simulink library "control_design_lib"  (Simulink 7.1)
libraries: control_design_lib x1
settings Model: Creator=jporter  LastModifiedBy=jporter

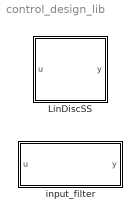
== system control_design_lib ==
  LinDiscSS : Subsystem  mask(Linear Discrete State Space){Add=0, Bdd=0, Cdd=0, Ddd=0, x0=0, Tsamp=0}
      mask prompts: Add "Ad"; Bdd "Bd"; Cdd "Cd"; Ddd "Dd"; x0 "Initial condition:"; Tsamp "Sample time:"
      mask help:
      | Implements a linear discrete state-space filter using blocks
      | which are compatible with the HCDDES toolchain code generator.
  input_filter : Subsystem  mask{wn=1, zeta=0.9, Tsamp=0.02}
      mask prompts: wn "omega_n"; Tsamp "Sample time"
      mask init:
      | Fsys = tf([wn^2],[1,2*zeta*wn,wn^2]);
      | Fd = c2d( Fsys, Tsamp, 'zoh' );
      | FS = ss( Fd );
      | Add = FS.a;
      | Bdd = FS.b;
      | Cdd = FS.c;
      | Ddd = FS.d;

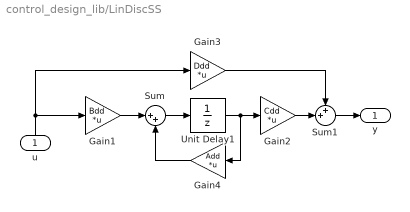
== system control_design_lib/LinDiscSS ==
  u : Inport  Orientation=up
  Gain1 : Gain  Gain=Bdd  Multiplication=Matrix(K*u)  ParameterDataType=sfix(16)  ParameterScaling=2^0  OutDataType=sfix(16)  OutScaling=2^0
  Gain2 : Gain  Gain=Cdd  Multiplication=Matrix(K*u) (u vector)  ParameterDataType=sfix(16)  ParameterScaling=2^0  OutDataType=sfix(16)  OutScaling=2^0
  Gain3 : Gain  Gain=Ddd  Multiplication=Matrix(K*u)  ParameterDataType=sfix(16)  ParameterScaling=2^0  OutDataType=sfix(16)  OutScaling=2^0
  Gain4 : Gain  Orientation=left  Gain=Add  Multiplication=Matrix(K*u) (u vector)  ParameterDataType=sfix(16)  ParameterScaling=2^0  OutDataType=sfix(16)  OutScaling=2^0
  Sum : Sum  Inputs=|++  OutDataType=sfix(16)  OutScaling=2^0
  Sum1 : Sum  Inputs=++|  OutDataType=sfix(16)  OutScaling=2^0
  Unit Delay1 : UnitDelay  X0=x0  SampleTime=Tsamp
  y : Outport
  wires:
  Gain1/1 -> Sum/1
  Gain3/1 -> Sum1/1
  Gain2/1 -> Sum1/2
  Sum/1 -> Unit Delay1/1
  Unit Delay1/1 -> Gain2/1, Gain4/1
  Gain4/1 -> Sum/2
  u/1 -> Gain1/1, Gain3/1
  Sum1/1 -> y/1

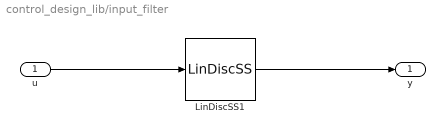
== system control_design_lib/input_filter ==
  u : Inport  OutDataType=sfix(16)  OutScaling=2^0
  LinDiscSS1 : control_design_lib/LinDiscSS  SystemSampleTime=-1  Add=Add  Bdd=Bdd  Cdd=Cdd  Ddd=Ddd  x0=[0 0]  Tsamp=Tsamp
  y : Outport  OutDataType=sfix(16)  OutScaling=2^0
  wires:
  u/1 -> LinDiscSS1/1
  LinDiscSS1/1 -> y/1
